simulink model "Filter"  (R2014a)
settings: Solver=FixedStepDiscrete  StartTime=0.0  StopTime=inf  FixedStep=SampleTime  RelTol=1e-3
values from neighbouring files (symbols this model uses):
  SampleTime = evalin('base','SampleTime')    [FIDF_Design.m]    (also in FIDF_Designing.m; FIDF_Framework.m; default_settings.m = 0.01; gui_main.m)
settings Model: Creator=georg  LastModifiedBy=Maik

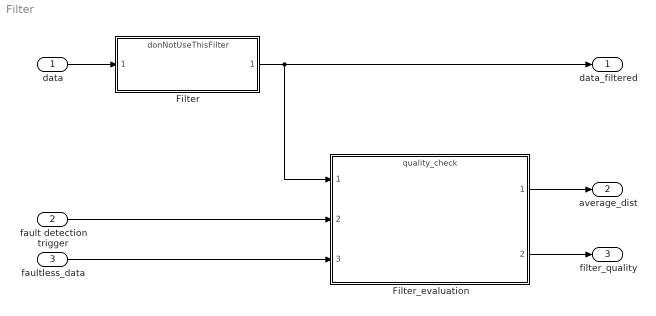
== system Filter ==
  data : Inport
  fault detection trigger : Inport  Port=2  OutDataTypeStr=Bus: TriggerBus  SampleTime=SampleTime
  faultless_data : Inport  Port=3
  Filter : ModelReference  ModelNameDialog=donNotUseThisFilter  SimulationMode=Normal  ModelReferenceVersion=1.6  DefaultDataLogging=on
  Filter_evaluation : ModelReference  ModelNameDialog=quality_check.slx  SimulationMode=Normal  ModelReferenceVersion=1.71  CopyOfModelName=quality_check.slx  DefaultDataLogging=on
  data_filtered : Outport
  average_dist : Outport  Port=2
  filter_quality : Outport  Port=3
  wires:
  data/1 -> Filter/1
  Filter/1 -> Filter_evaluation/1, data_filtered/1
  faultless_data/1 -> Filter_evaluation/3
  fault detection trigger/1 -> Filter_evaluation/2
  Filter_evaluation/1 -> average_dist/1
  Filter_evaluation/2 -> filter_quality/1
